simulink library "MBDS_Subsystems"  (R2018b)
settings: Solver=ode45  StartTime=0.0  StopTime=10.0  RelTol=1e-3
undefined symbols (not defined in the file or in its folder): nbo_False, nbo_True
libraries: KIBES_Signal x1438, MBDS_Modules x44, simulink x2
(part 8 of 15)

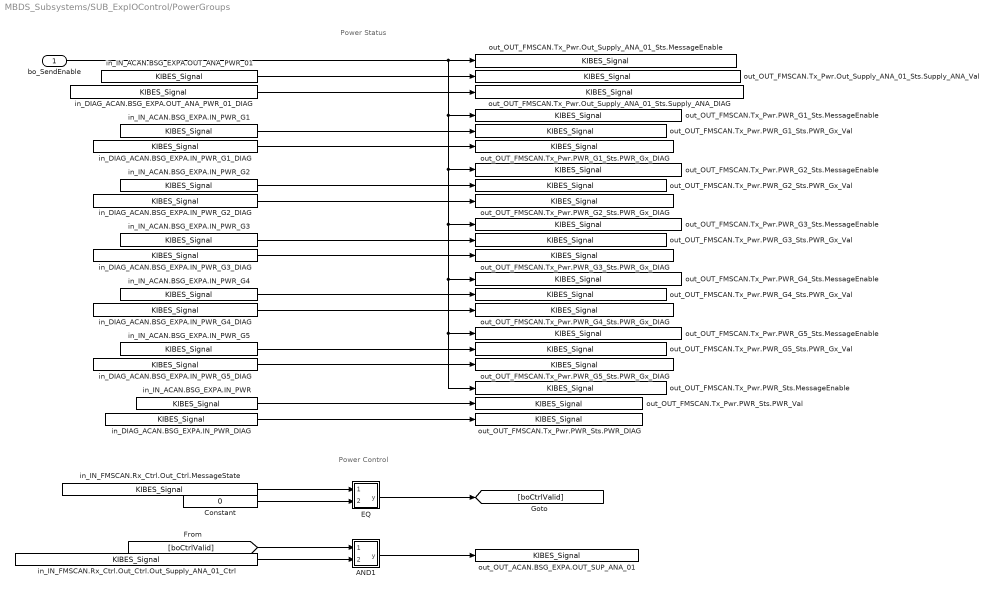
== system MBDS_Subsystems/SUB_ExpIOControl/PowerGroups ==
  note: Power Control
  note: Power Status
  bo_SendEnable : Inport
  AND1 : Subsystem  InitFcn=|  mask(AND){MBDS_LibraryBlock=on, BitwiseMode=off, Inputs=2, UseBitMask=off, BitMask='A7', OutDataTypeStr=Inherit: Inherit via back propagation, MBDS_BlockVersion=08.20.02}
      | if(exist('MBDS_BlockCallback', 'file'))
      |    MBDS_BlockCallback('Update', gcb);
      | end
      mask prompts: MBDS_LibraryBlock "MBDS library block"; BitwiseMode "Use 'bitwise' mode"; Inputs "Number of input ports:"; UseBitMask "Use bit mask"; BitMask "Bit mask:"; OutDataTypeStr "Output data type:"; MBDS_BlockVersion "Version:"
      mask help: Logical or bitwise AND operator. For multiple inputs, operators are applied across the inputs. For a single input, operators are applied across the input vector. In bitwise mode a bit mask can be applied onto single input signals.
      mask init: same as MBDS_Subsystems/SUB_DateTime/AND
      mask Help: eval(['open([workdir(''library_dir:''),''\Blockset\help\'',get_param(gcb,''MaskType''),''.html''])'])
      mask Callback BitwiseMode:
      | if(exist('MBDS_BlockCallback', 'file'))
      |    MBDS_BlockCallback('BitwiseMode', gcb);
      | end
      mask Callback Inputs:
      | if(exist('MBDS_BlockCallback', 'file'))
      |    MBDS_BlockCallback('Inputs', gcb);
      | end
      mask Callback UseBitMask:
      | if(exist('MBDS_BlockCallback', 'file'))
      |    MBDS_BlockCallback('UseBitMask', gcb);
      | end
      mask Callback BitMask:
      | if(exist('MBDS_BlockCallback', 'file'))
      |    MBDS_BlockCallback('BitMask', gcb);
      | end
      mask TypeOptions OutDataTypeStr: Inherit: Inherit via back propagation | int8 | uint8 | int16 | uint16 | int32 | uint32 | boolean
      mask Callback OutDataTypeStr:
      | % Adopt Value
      | if(exist('MBDS_BlockCallback', 'file'))
      |    MBDS_BlockCallback('OutDataTypeStr', gcb);
      | end
      mask DialogControl ParameterTabVar0 Prompt: Main
      mask DialogControl ParameterTabVar01 Prompt: Signal Attributes
      mask DialogControl ParameterTabVar012 Prompt: Version
      mask Display:
      | % Show icon or block text
      | if(UseBitMask)
      |    if(isnumeric(BitMask))
      |       BitMaskString = ['0x',dec2hex(floor(BitMask))];
      |    elseif(ischar(BitMask))
      |       BitMaskString = ['0x',upper(BitMask)];
      |    else
      |       BitMaskString = '???';
      |    end
      |    disp(sprintf(['AND\n', BitMaskString]))
      | else
      |    disp('AND')
      | end
  Constant : Constant  InitFcn=|  Value=0  OutDataTypeStr=uint16
      | if(exist('MBDS_BlockCallback', 'file'))
      |    MBDS_BlockCallback('Update', gcb);  
      | end
  EQ : Subsystem  InitFcn=|  mask(EQ){MBDS_LibraryBlock=on, InputSameDT=on, MBDS_BlockVersion=08.20.02}
      | if(exist('MBDS_BlockCallback', 'file'))
      |    MBDS_BlockCallback('Update', gcb);
      | end
      mask prompts: MBDS_LibraryBlock "MBDS library block"; InputSameDT "Require all inputs to have the same data type"; MBDS_BlockVersion "Block version:"
      mask help: The block compares if both input signals are equal.
      mask init: same as MBDS_Subsystems/SUB_DateTime/AND
      mask Help: eval(['open([workdir(''library_dir:''),''\Blockset\help\'',get_param(gcb,''MaskType''),''.html''])'])
      mask Callback InputSameDT:
      | % Adopt value
      | if(exist('MBDS_BlockCallback', 'file'))
      |    MBDS_BlockCallback('InputSameDT', gcb);
      | end
      mask DialogControl ParameterTabVar0 Prompt: Signal Attributes
      mask DialogControl ParameterTabVar01 Prompt: Version
      mask Display:
      | % Show icon or block text
      | if(exist('MBDS_BlockCallback', 'file'))
      |    image(imread('EQ.tif','tif'),[0.35,0.35,0.355,0.25])
      |    disp('')
      | else
      |    disp(sprintf('=='));
      | end
  in_DIAG_ACAN.BSG_EXPA.IN_PWR_DIAG : KIBES_Signal/KIBES_Signal  MBDS_LibraryBlock=on  DatabaseKey=837  SignalName=DIAG_ACAN.BSG_EXPA.IN_PWR_DIAG  SymbolName=DIAG_ACAN_BSG_EXPA_IN_PWR_DIAG_000837  DataType=uint16  Init=1  Slope=1  Bias=0  DataSize=1  fpDataType=uint16  BlockIOType=Inport  DeviceType=0
  in_DIAG_ACAN.BSG_EXPA.IN_PWR_G1_DIAG : KIBES_Signal/KIBES_Signal  MBDS_LibraryBlock=on  DatabaseKey=835  SignalName=DIAG_ACAN.BSG_EXPA.IN_PWR_G1_DIAG  SymbolName=DIAG_ACAN_BSG_EXPA_IN_PWR_G1_DIAG_000835  DataType=uint16  Init=1  Slope=1  Bias=0  DataSize=1  fpDataType=uint16  BlockIOType=Inport  DeviceType=0
  in_DIAG_ACAN.BSG_EXPA.IN_PWR_G2_DIAG : KIBES_Signal/KIBES_Signal  MBDS_LibraryBlock=on  DatabaseKey=830  SignalName=DIAG_ACAN.BSG_EXPA.IN_PWR_G2_DIAG  SymbolName=DIAG_ACAN_BSG_EXPA_IN_PWR_G2_DIAG_000830  DataType=uint16  Init=1  Slope=1  Bias=0  DataSize=1  fpDataType=uint16  BlockIOType=Inport  DeviceType=0
  in_DIAG_ACAN.BSG_EXPA.IN_PWR_G3_DIAG : KIBES_Signal/KIBES_Signal  MBDS_LibraryBlock=on  DatabaseKey=833  SignalName=DIAG_ACAN.BSG_EXPA.IN_PWR_G3_DIAG  SymbolName=DIAG_ACAN_BSG_EXPA_IN_PWR_G3_DIAG_000833  DataType=uint16  Init=1  Slope=1  Bias=0  DataSize=1  fpDataType=uint16  BlockIOType=Inport  DeviceType=0
  in_DIAG_ACAN.BSG_EXPA.IN_PWR_G4_DIAG : KIBES_Signal/KIBES_Signal  MBDS_LibraryBlock=on  DatabaseKey=832  SignalName=DIAG_ACAN.BSG_EXPA.IN_PWR_G4_DIAG  SymbolName=DIAG_ACAN_BSG_EXPA_IN_PWR_G4_DIAG_000832  DataType=uint16  Init=1  Slope=1  Bias=0  DataSize=1  fpDataType=uint16  BlockIOType=Inport  DeviceType=0
  in_DIAG_ACAN.BSG_EXPA.IN_PWR_G5_DIAG : KIBES_Signal/KIBES_Signal  MBDS_LibraryBlock=on  DatabaseKey=834  SignalName=DIAG_ACAN.BSG_EXPA.IN_PWR_G5_DIAG  SymbolName=DIAG_ACAN_BSG_EXPA_IN_PWR_G5_DIAG_000834  DataType=uint16  Init=1  Slope=1  Bias=0  DataSize=1  fpDataType=uint16  BlockIOType=Inport  DeviceType=0
  in_DIAG_ACAN.BSG_EXPA.OUT_ANA_PWR_01_DIAG : KIBES_Signal/KIBES_Signal  MBDS_LibraryBlock=on  DatabaseKey=813  SignalName=DIAG_ACAN.BSG_EXPA.OUT_ANA_PWR_01_DIAG  SymbolName=DIAG_ACAN_BSG_EXPA_OUT_ANA_PWR_01_DIAG_000813  DataType=uint16  Init=1  Slope=1  Bias=0  DataSize=1  fpDataType=uint16  BlockIOType=Inport  DeviceType=0
  in_IN_ACAN.BSG_EXPA.IN_PWR : KIBES_Signal/KIBES_Signal  MBDS_LibraryBlock=on  DatabaseKey=838  SignalName=IN_ACAN.BSG_EXPA.IN_PWR  SymbolName=IN_ACAN_BSG_EXPA_IN_PWR_000838  DataType=uint32  Init=0  Slope=1  Bias=0  DataSize=1  fpDataType=uint32  BlockIOType=Inport  DeviceType=0
  in_IN_ACAN.BSG_EXPA.IN_PWR_G1 : KIBES_Signal/KIBES_Signal  MBDS_LibraryBlock=on  DatabaseKey=836  SignalName=IN_ACAN.BSG_EXPA.IN_PWR_G1  SymbolName=IN_ACAN_BSG_EXPA_IN_PWR_G1_000836  DataType=uint16  Init=0  Slope=1  Bias=0  DataSize=1  fpDataType=uint16  BlockIOType=Inport  DeviceType=0
  in_IN_ACAN.BSG_EXPA.IN_PWR_G2 : KIBES_Signal/KIBES_Signal  MBDS_LibraryBlock=on  DatabaseKey=840  SignalName=IN_ACAN.BSG_EXPA.IN_PWR_G2  SymbolName=IN_ACAN_BSG_EXPA_IN_PWR_G2_000840  DataType=uint16  Init=0  Slope=1  Bias=0  DataSize=1  fpDataType=uint16  BlockIOType=Inport  DeviceType=0
  in_IN_ACAN.BSG_EXPA.IN_PWR_G3 : KIBES_Signal/KIBES_Signal  MBDS_LibraryBlock=on  DatabaseKey=829  SignalName=IN_ACAN.BSG_EXPA.IN_PWR_G3  SymbolName=IN_ACAN_BSG_EXPA_IN_PWR_G3_000829  DataType=uint16  Init=0  Slope=1  Bias=0  DataSize=1  fpDataType=uint16  BlockIOType=Inport  DeviceType=0
  in_IN_ACAN.BSG_EXPA.IN_PWR_G4 : KIBES_Signal/KIBES_Signal  MBDS_LibraryBlock=on  DatabaseKey=839  SignalName=IN_ACAN.BSG_EXPA.IN_PWR_G4  SymbolName=IN_ACAN_BSG_EXPA_IN_PWR_G4_000839  DataType=uint16  Init=0  Slope=1  Bias=0  DataSize=1  fpDataType=uint16  BlockIOType=Inport  DeviceType=0
  in_IN_ACAN.BSG_EXPA.IN_PWR_G5 : KIBES_Signal/KIBES_Signal  MBDS_LibraryBlock=on  DatabaseKey=831  SignalName=IN_ACAN.BSG_EXPA.IN_PWR_G5  SymbolName=IN_ACAN_BSG_EXPA_IN_PWR_G5_000831  DataType=uint16  Init=0  Slope=1  Bias=0  DataSize=1  fpDataType=uint16  BlockIOType=Inport  DeviceType=0
  in_IN_ACAN.BSG_EXPA.OUT_ANA_PWR_01 : KIBES_Signal/KIBES_Signal  MBDS_LibraryBlock=on  DatabaseKey=810  SignalName=IN_ACAN.BSG_EXPA.OUT_ANA_PWR_01  SymbolName=IN_ACAN_BSG_EXPA_OUT_ANA_PWR_01_000810  DataType=uint16  Init=0  Slope=1  Bias=0  DataSize=1  fpDataType=uint16  BlockIOType=Inport  DeviceType=0
  in_IN_FMSCAN.Rx_Ctrl.Out_Ctrl.MessageState : KIBES_Signal/KIBES_Signal  MBDS_LibraryBlock=on  DatabaseKey=2678  SignalName=IN_FMSCAN.Rx_Ctrl.Out_Ctrl.MessageState  SymbolName=IN_FMSCAN_Rx_Ctrl_Out_Ctrl_MessageState_002678  DataType=uint16  Init=0  Slope=1  Bias=0  DataSize=1  fpDataType=uint16  BlockIOType=Inport  DeviceType=0
  in_IN_FMSCAN.Rx_Ctrl.Out_Ctrl.Out_Supply_ANA_01_Ctrl : KIBES_Signal/KIBES_Signal  MBDS_LibraryBlock=on  DatabaseKey=2663  SignalName=IN_FMSCAN.Rx_Ctrl.Out_Ctrl.Out_Supply_ANA_01_Ctrl  SymbolName=IN_FMSCAN_Rx_Ctrl_Out_Ctrl_Out_Supply_ANA_01_Ctrl_002663  DataType=boolean  Init=0  Slope=1  Bias=0  DataSize=1  fpDataType=boolean  BlockIOType=Inport  DeviceType=0
  out_OUT_ACAN.BSG_EXPA.OUT_SUP_ANA_01 : KIBES_Signal/KIBES_Signal  MBDS_LibraryBlock=on  DatabaseKey=933  SignalName=OUT_ACAN.BSG_EXPA.OUT_SUP_ANA_01  SymbolName=OUT_ACAN_BSG_EXPA_OUT_SUP_ANA_01_000933  DataType=boolean  Init=0  Slope=1  Bias=0  DataSize=1  fpDataType=boolean  BlockIOType=Outport  DeviceType=0
  out_OUT_FMSCAN.Tx_Pwr.Out_Supply_ANA_01_Sts.MessageEnable : KIBES_Signal/KIBES_Signal  MBDS_LibraryBlock=on  DatabaseKey=2629  SignalName=OUT_FMSCAN.Tx_Pwr.Out_Supply_ANA_01_Sts.MessageEnable  SymbolName=OUT_FMSCAN_Tx_Pwr_Out_Supply_ANA_01_Sts_MessageEnable_002629  DataType=boolean  Init=0  Slope=1  Bias=0  DataSize=1  fpDataType=boolean  BlockIOType=Outport  DeviceType=0
  out_OUT_FMSCAN.Tx_Pwr.Out_Supply_ANA_01_Sts.Supply_ANA_DIAG : KIBES_Signal/KIBES_Signal  MBDS_LibraryBlock=on  DatabaseKey=2615  SignalName=OUT_FMSCAN.Tx_Pwr.Out_Supply_ANA_01_Sts.Supply_ANA_DIAG  SymbolName=OUT_FMSCAN_Tx_Pwr_Out_Supply_ANA_01_Sts_Supply_ANA_DIAG_002615  DataType=uint16  Init=0  Slope=1  Bias=0  DataSize=1  fpDataType=uint16  BlockIOType=Outport  DeviceType=0
  out_OUT_FMSCAN.Tx_Pwr.Out_Supply_ANA_01_Sts.Supply_ANA_Val : KIBES_Signal/KIBES_Signal  MBDS_LibraryBlock=on  DatabaseKey=2616  SignalName=OUT_FMSCAN.Tx_Pwr.Out_Supply_ANA_01_Sts.Supply_ANA_Val  SymbolName=OUT_FMSCAN_Tx_Pwr_Out_Supply_ANA_01_Sts_Supply_ANA_Val_002616  DataType=uint16  Init=0  Slope=1  Bias=0  DataSize=1  fpDataType=uint16  BlockIOType=Outport  DeviceType=0
  out_OUT_FMSCAN.Tx_Pwr.PWR_G1_Sts.MessageEnable : KIBES_Signal/KIBES_Signal  MBDS_LibraryBlock=on  DatabaseKey=2630  SignalName=OUT_FMSCAN.Tx_Pwr.PWR_G1_Sts.MessageEnable  SymbolName=OUT_FMSCAN_Tx_Pwr_PWR_G1_Sts_MessageEnable_002630  DataType=boolean  Init=0  Slope=1  Bias=0  DataSize=1  fpDataType=boolean  BlockIOType=Outport  DeviceType=0
  out_OUT_FMSCAN.Tx_Pwr.PWR_G1_Sts.PWR_Gx_DIAG : KIBES_Signal/KIBES_Signal  MBDS_LibraryBlock=on  DatabaseKey=2617  SignalName=OUT_FMSCAN.Tx_Pwr.PWR_G1_Sts.PWR_Gx_DIAG  SymbolName=OUT_FMSCAN_Tx_Pwr_PWR_G1_Sts_PWR_Gx_DIAG_002617  DataType=uint16  Init=0  Slope=1  Bias=0  DataSize=1  fpDataType=uint16  BlockIOType=Outport  DeviceType=0
  out_OUT_FMSCAN.Tx_Pwr.PWR_G1_Sts.PWR_Gx_Val : KIBES_Signal/KIBES_Signal  MBDS_LibraryBlock=on  DatabaseKey=2618  SignalName=OUT_FMSCAN.Tx_Pwr.PWR_G1_Sts.PWR_Gx_Val  SymbolName=OUT_FMSCAN_Tx_Pwr_PWR_G1_Sts_PWR_Gx_Val_002618  DataType=uint16  Init=0  Slope=1  Bias=0  DataSize=1  fpDataType=uint16  BlockIOType=Outport  DeviceType=0
  out_OUT_FMSCAN.Tx_Pwr.PWR_G2_Sts.MessageEnable : KIBES_Signal/KIBES_Signal  MBDS_LibraryBlock=on  DatabaseKey=2631  SignalName=OUT_FMSCAN.Tx_Pwr.PWR_G2_Sts.MessageEnable  SymbolName=OUT_FMSCAN_Tx_Pwr_PWR_G2_Sts_MessageEnable_002631  DataType=boolean  Init=0  Slope=1  Bias=0  DataSize=1  fpDataType=boolean  BlockIOType=Outport  DeviceType=0
  out_OUT_FMSCAN.Tx_Pwr.PWR_G2_Sts.PWR_Gx_DIAG : KIBES_Signal/KIBES_Signal  MBDS_LibraryBlock=on  DatabaseKey=2619  SignalName=OUT_FMSCAN.Tx_Pwr.PWR_G2_Sts.PWR_Gx_DIAG  SymbolName=OUT_FMSCAN_Tx_Pwr_PWR_G2_Sts_PWR_Gx_DIAG_002619  DataType=uint16  Init=0  Slope=1  Bias=0  DataSize=1  fpDataType=uint16  BlockIOType=Outport  DeviceType=0
  out_OUT_FMSCAN.Tx_Pwr.PWR_G2_Sts.PWR_Gx_Val : KIBES_Signal/KIBES_Signal  MBDS_LibraryBlock=on  DatabaseKey=2620  SignalName=OUT_FMSCAN.Tx_Pwr.PWR_G2_Sts.PWR_Gx_Val  SymbolName=OUT_FMSCAN_Tx_Pwr_PWR_G2_Sts_PWR_Gx_Val_002620  DataType=uint16  Init=0  Slope=1  Bias=0  DataSize=1  fpDataType=uint16  BlockIOType=Outport  DeviceType=0
  out_OUT_FMSCAN.Tx_Pwr.PWR_G3_Sts.MessageEnable : KIBES_Signal/KIBES_Signal  MBDS_LibraryBlock=on  DatabaseKey=2632  SignalName=OUT_FMSCAN.Tx_Pwr.PWR_G3_Sts.MessageEnable  SymbolName=OUT_FMSCAN_Tx_Pwr_PWR_G3_Sts_MessageEnable_002632  DataType=boolean  Init=0  Slope=1  Bias=0  DataSize=1  fpDataType=boolean  BlockIOType=Outport  DeviceType=0
  out_OUT_FMSCAN.Tx_Pwr.PWR_G3_Sts.PWR_Gx_DIAG : KIBES_Signal/KIBES_Signal  MBDS_LibraryBlock=on  DatabaseKey=2621  SignalName=OUT_FMSCAN.Tx_Pwr.PWR_G3_Sts.PWR_Gx_DIAG  SymbolName=OUT_FMSCAN_Tx_Pwr_PWR_G3_Sts_PWR_Gx_DIAG_002621  DataType=uint16  Init=0  Slope=1  Bias=0  DataSize=1  fpDataType=uint16  BlockIOType=Outport  DeviceType=0
  out_OUT_FMSCAN.Tx_Pwr.PWR_G3_Sts.PWR_Gx_Val : KIBES_Signal/KIBES_Signal  MBDS_LibraryBlock=on  DatabaseKey=2622  SignalName=OUT_FMSCAN.Tx_Pwr.PWR_G3_Sts.PWR_Gx_Val  SymbolName=OUT_FMSCAN_Tx_Pwr_PWR_G3_Sts_PWR_Gx_Val_002622  DataType=uint16  Init=0  Slope=1  Bias=0  DataSize=1  fpDataType=uint16  BlockIOType=Outport  DeviceType=0
  out_OUT_FMSCAN.Tx_Pwr.PWR_G4_Sts.MessageEnable : KIBES_Signal/KIBES_Signal  MBDS_LibraryBlock=on  DatabaseKey=2633  SignalName=OUT_FMSCAN.Tx_Pwr.PWR_G4_Sts.MessageEnable  SymbolName=OUT_FMSCAN_Tx_Pwr_PWR_G4_Sts_MessageEnable_002633  DataType=boolean  Init=0  Slope=1  Bias=0  DataSize=1  fpDataType=boolean  BlockIOType=Outport  DeviceType=0
  out_OUT_FMSCAN.Tx_Pwr.PWR_G4_Sts.PWR_Gx_DIAG : KIBES_Signal/KIBES_Signal  MBDS_LibraryBlock=on  DatabaseKey=2623  SignalName=OUT_FMSCAN.Tx_Pwr.PWR_G4_Sts.PWR_Gx_DIAG  SymbolName=OUT_FMSCAN_Tx_Pwr_PWR_G4_Sts_PWR_Gx_DIAG_002623  DataType=uint16  Init=0  Slope=1  Bias=0  DataSize=1  fpDataType=uint16  BlockIOType=Outport  DeviceType=0
  out_OUT_FMSCAN.Tx_Pwr.PWR_G4_Sts.PWR_Gx_Val : KIBES_Signal/KIBES_Signal  MBDS_LibraryBlock=on  DatabaseKey=2624  SignalName=OUT_FMSCAN.Tx_Pwr.PWR_G4_Sts.PWR_Gx_Val  SymbolName=OUT_FMSCAN_Tx_Pwr_PWR_G4_Sts_PWR_Gx_Val_002624  DataType=uint16  Init=0  Slope=1  Bias=0  DataSize=1  fpDataType=uint16  BlockIOType=Outport  DeviceType=0
  out_OUT_FMSCAN.Tx_Pwr.PWR_G5_Sts.MessageEnable : KIBES_Signal/KIBES_Signal  MBDS_LibraryBlock=on  DatabaseKey=2634  SignalName=OUT_FMSCAN.Tx_Pwr.PWR_G5_Sts.MessageEnable  SymbolName=OUT_FMSCAN_Tx_Pwr_PWR_G5_Sts_MessageEnable_002634  DataType=boolean  Init=0  Slope=1  Bias=0  DataSize=1  fpDataType=boolean  BlockIOType=Outport  DeviceType=0
  out_OUT_FMSCAN.Tx_Pwr.PWR_G5_Sts.PWR_Gx_DIAG : KIBES_Signal/KIBES_Signal  MBDS_LibraryBlock=on  DatabaseKey=2625  SignalName=OUT_FMSCAN.Tx_Pwr.PWR_G5_Sts.PWR_Gx_DIAG  SymbolName=OUT_FMSCAN_Tx_Pwr_PWR_G5_Sts_PWR_Gx_DIAG_002625  DataType=uint16  Init=0  Slope=1  Bias=0  DataSize=1  fpDataType=uint16  BlockIOType=Outport  DeviceType=0
  out_OUT_FMSCAN.Tx_Pwr.PWR_G5_Sts.PWR_Gx_Val : KIBES_Signal/KIBES_Signal  MBDS_LibraryBlock=on  DatabaseKey=2626  SignalName=OUT_FMSCAN.Tx_Pwr.PWR_G5_Sts.PWR_Gx_Val  SymbolName=OUT_FMSCAN_Tx_Pwr_PWR_G5_Sts_PWR_Gx_Val_002626  DataType=uint16  Init=0  Slope=1  Bias=0  DataSize=1  fpDataType=uint16  BlockIOType=Outport  DeviceType=0
  out_OUT_FMSCAN.Tx_Pwr.PWR_Sts.MessageEnable : KIBES_Signal/KIBES_Signal  MBDS_LibraryBlock=on  DatabaseKey=2635  SignalName=OUT_FMSCAN.Tx_Pwr.PWR_Sts.MessageEnable  SymbolName=OUT_FMSCAN_Tx_Pwr_PWR_Sts_MessageEnable_002635  DataType=boolean  Init=0  Slope=1  Bias=0  DataSize=1  fpDataType=boolean  BlockIOType=Outport  DeviceType=0
  out_OUT_FMSCAN.Tx_Pwr.PWR_Sts.PWR_DIAG : KIBES_Signal/KIBES_Signal  MBDS_LibraryBlock=on  DatabaseKey=2627  SignalName=OUT_FMSCAN.Tx_Pwr.PWR_Sts.PWR_DIAG  SymbolName=OUT_FMSCAN_Tx_Pwr_PWR_Sts_PWR_DIAG_002627  DataType=uint16  Init=0  Slope=1  Bias=0  DataSize=1  fpDataType=uint16  BlockIOType=Outport  DeviceType=0
  out_OUT_FMSCAN.Tx_Pwr.PWR_Sts.PWR_Val : KIBES_Signal/KIBES_Signal  MBDS_LibraryBlock=on  DatabaseKey=2628  SignalName=OUT_FMSCAN.Tx_Pwr.PWR_Sts.PWR_Val  SymbolName=OUT_FMSCAN_Tx_Pwr_PWR_Sts_PWR_Val_002628  DataType=uint32  Init=0  Slope=1  Bias=0  DataSize=1  fpDataType=uint32  BlockIOType=Outport  DeviceType=0
  wires:
  AND1/1(y) -> out_OUT_ACAN.BSG_EXPA.OUT_SUP_ANA_01/1
  in_IN_FMSCAN.Rx_Ctrl.Out_Ctrl.Out_Supply_ANA_01_Ctrl/1 -> AND1/2(u2)
  [boCtrlValid] -> AND1/1(u1)
  EQ/1(y) -> [boCtrlValid]
  Constant/1 -> EQ/2(u2)
  in_IN_FMSCAN.Rx_Ctrl.Out_Ctrl.MessageState/1 -> EQ/1(u1)
  in_IN_ACAN.BSG_EXPA.OUT_ANA_PWR_01/1 -> out_OUT_FMSCAN.Tx_Pwr.Out_Supply_ANA_01_Sts.Supply_ANA_Val/1
  in_DIAG_ACAN.BSG_EXPA.IN_PWR_DIAG/1 -> out_OUT_FMSCAN.Tx_Pwr.PWR_Sts.PWR_DIAG/1
  in_IN_ACAN.BSG_EXPA.IN_PWR_G5/1 -> out_OUT_FMSCAN.Tx_Pwr.PWR_G5_Sts.PWR_Gx_Val/1
  in_DIAG_ACAN.BSG_EXPA.IN_PWR_G5_DIAG/1 -> out_OUT_FMSCAN.Tx_Pwr.PWR_G5_Sts.PWR_Gx_DIAG/1
  in_IN_ACAN.BSG_EXPA.IN_PWR_G4/1 -> out_OUT_FMSCAN.Tx_Pwr.PWR_G4_Sts.PWR_Gx_Val/1
  in_DIAG_ACAN.BSG_EXPA.IN_PWR_G4_DIAG/1 -> out_OUT_FMSCAN.Tx_Pwr.PWR_G4_Sts.PWR_Gx_DIAG/1
  in_DIAG_ACAN.BSG_EXPA.IN_PWR_G1_DIAG/1 -> out_OUT_FMSCAN.Tx_Pwr.PWR_G1_Sts.PWR_Gx_DIAG/1
  in_IN_ACAN.BSG_EXPA.IN_PWR_G3/1 -> out_OUT_FMSCAN.Tx_Pwr.PWR_G3_Sts.PWR_Gx_Val/1
  in_IN_ACAN.BSG_EXPA.IN_PWR_G2/1 -> out_OUT_FMSCAN.Tx_Pwr.PWR_G2_Sts.PWR_Gx_Val/1
  bo_SendEnable/1 -> out_OUT_FMSCAN.Tx_Pwr.PWR_G5_Sts.MessageEnable/1, out_OUT_FMSCAN.Tx_Pwr.PWR_Sts.MessageEnable/1, out_OUT_FMSCAN.Tx_Pwr.PWR_G4_Sts.MessageEnable/1, out_OUT_FMSCAN.Tx_Pwr.PWR_G3_Sts.MessageEnable/1, out_OUT_FMSCAN.Tx_Pwr.PWR_G2_Sts.MessageEnable/1, out_OUT_FMSCAN.Tx_Pwr.PWR_G1_Sts.MessageEnable/1, out_OUT_FMSCAN.Tx_Pwr.Out_Supply_ANA_01_Sts.MessageEnable/1
  in_IN_ACAN.BSG_EXPA.IN_PWR/1 -> out_OUT_FMSCAN.Tx_Pwr.PWR_Sts.PWR_Val/1
  in_DIAG_ACAN.BSG_EXPA.IN_PWR_G2_DIAG/1 -> out_OUT_FMSCAN.Tx_Pwr.PWR_G2_Sts.PWR_Gx_DIAG/1
  in_IN_ACAN.BSG_EXPA.IN_PWR_G1/1 -> out_OUT_FMSCAN.Tx_Pwr.PWR_G1_Sts.PWR_Gx_Val/1
  in_DIAG_ACAN.BSG_EXPA.IN_PWR_G3_DIAG/1 -> out_OUT_FMSCAN.Tx_Pwr.PWR_G3_Sts.PWR_Gx_DIAG/1
  in_DIAG_ACAN.BSG_EXPA.OUT_ANA_PWR_01_DIAG/1 -> out_OUT_FMSCAN.Tx_Pwr.Out_Supply_ANA_01_Sts.Supply_ANA_DIAG/1
